simulink subsystem "motor_pos"  (R2020a)
settings: Solver=VariableStepAuto  StartTime=0.0  StopTime=10.0  RelTol=1e-3
values from neighbouring files (symbols this model uses):
  b = 3.5076999999999995E-6    [data.sldd]    (also in para4.m = 3.5077e-06)
  J = 3.2280000000000003E-6    [data.sldd]    (also in para4.m = 3.228e-06)
  ke = 0.0274    [data.sldd]    (also in para4.m)
  kt = 0.0274    [data.sldd]    (also in para4.m)
  L = 2.75E-6    [data.sldd]    (also in para4.m = 2.75e-06)
  R = 4.0    [data.sldd]    (also in para4.m = 4)
settings Model: Creator=vijay  LastModifiedBy=vijay

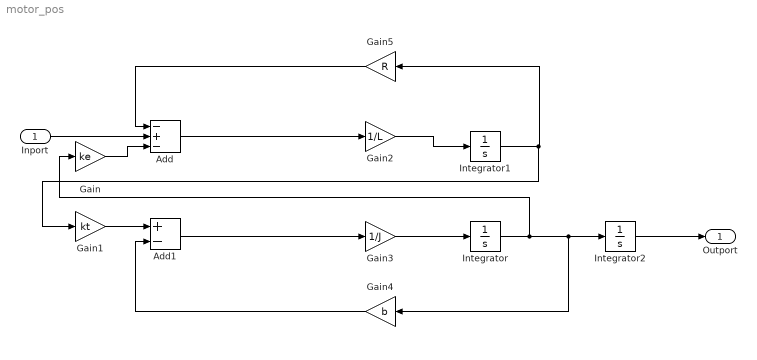
== system motor_pos ==
  Inport : Inport
  Add : Sum  Inputs=-+-
  Add1 : Sum  Inputs=+-
  Gain : Gain  Gain=ke
  Gain1 : Gain  Gain=kt
  Gain2 : Gain  Gain=1/L
  Gain3 : Gain  Gain=1/J
  Gain4 : Gain  Gain=b
  Gain5 : Gain  Gain=R
  Integrator : Integrator
  Integrator1 : Integrator
  Integrator2 : Integrator
  Outport : Outport
  wires:
  Integrator/1 -> Integrator2/1, Gain4/1, Gain/1
  Gain5/1 -> Add/1
  Gain3/1 -> Integrator/1
  Integrator1/1 -> Gain5/1, Gain1/1
  Inport/1 -> Add/2
  Gain/1 -> Add/3
  Gain1/1 -> Add1/1
  Integrator2/1 -> Outport/1
  Gain4/1 -> Add1/2
  Gain2/1 -> Integrator1/1
  Add1/1 -> Gain3/1
  Add/1 -> Gain2/1
